simulink model "single_phase_multilevel"  (R2025a)
settings: Solver=ode1be  StartTime=0.0  StopTime=simlength  FixedStep=tc  RelTol=1e-3
values from neighbouring files (symbols this model uses):
  Vfc1_base = Udc/5    [plotting_results.m]    (also in plotting_results_hf.m)
  Vfc2_base = 2*Vfc1_base    [plotting_results.m]    (also in plotting_results_hf.m)
  Vfc3_base = 3*Vfc1_base    [plotting_results.m]    (also in plotting_results_hf.m)
  Vfc4_base = 4*Vfc1_base    [plotting_results.m]    (also in plotting_results_hf.m)
undefined symbols (not defined in the file or in its folder): DThs_init, g0_4Hz, g1_4Hz, I_FS, kalman_omega, kalman_theta, ki_i_inv, ki_v_inv, kp_i_inv, kp_v_inv, Lconn, LFu1, m_dead_time, m_duty_open_loop, magnitude, n1, n10, omega_ref, phase_shift_mod11, phase_shift_mod21, phase_shift_mod31, phase_shift_mod41, phase_shift_mod51, precharge_off, q1kalman, q2kalman, Rbalance, Rconn, RFu, Rg_off, Rg_on, Rkalman, RLFu1, Rprecharge, Tambient, tc, time_pwm_enable, tPWM, ts, V_FS, VCFc_5_init, Vgate_base, weigth
libraries: fl_lib x281, nesl_utility x97, ee_lib x15, simulink x1
(part 2 of 6)

== system single_phase_multilevel/flying_capacitor_leg/fc1 ==
  CFc_1 : fl_lib/Electrical/Electrical Elements/Capacitor  c=CFc_1 F  r=1e-6 Ohm  g=0 1/Ohm  i_specify=off  i_priority=None  i=0 A  i_nominal_specify=off  i_nominal_value=1  i_nominal_unit=A  v_specify=off  v_priority=None  v=0 V  v_nominal_specify=off  v_nominal_value=1  v_nominal_unit=V  vc_specify=on  vc_priority=High  vc=VCFc_1_init V  vc_nominal_specify=off  vc_nominal_value=1  vc_nominal_unit=V
  CFi_HF_1 : fl_lib/Electrical/Electrical Elements/Capacitor  c=CFi_HF_1 F  r=1e-6 Ohm  g=0 1/Ohm  i_specify=off  i_priority=None  i=0 A  i_nominal_specify=off  i_nominal_value=1  i_nominal_unit=A  v_specify=off  v_priority=None  v=0 V  v_nominal_specify=off  v_nominal_value=1  v_nominal_unit=V  vc_specify=on  vc_priority=High  vc=VCFc_1_init V  vc_nominal_specify=off  vc_nominal_value=1  vc_nominal_unit=V
  Current Sensor : fl_lib/Electrical/Electrical Sensors/Current Sensor
  Current Sensor1 : fl_lib/Electrical/Electrical Sensors/Current Sensor
  LCFc_1 : fl_lib/Electrical/Electrical Elements/Inductor  l=LCFc_1 H  r=RCFc_1 Ohm  g=1e-9 1/Ohm  i_specify=off  i_priority=None  i=0 A  i_nominal_specify=off  i_nominal_value=1  i_nominal_unit=A  v_specify=off  v_priority=None  v=0 V  v_nominal_specify=off  v_nominal_value=1  v_nominal_unit=V  i_L_specify=off  i_L_priority=High  i_L=0 A  i_L_nominal_specify=off  i_L_nominal_value=1  i_L_nominal_unit=A
  LCFi_HF_1 : fl_lib/Electrical/Electrical Elements/Inductor  l=LCFi_HF_1 H  r=RCFi_HF_1 Ohm  g=1e-9 1/Ohm  i_specify=off  i_priority=None  i=0 A  i_nominal_specify=off  i_nominal_value=1  i_nominal_unit=A  v_specify=off  v_priority=None  v=0 V  v_nominal_specify=off  v_nominal_value=1  v_nominal_unit=V  i_L_specify=off  i_L_priority=High  i_L=0 A  i_L_nominal_specify=off  i_L_nominal_value=1  i_L_nominal_unit=A
  PS-Simulink Converter : nesl_utility/PS-Simulink Converter  PhysicalDomain=network_engine_domain  SubClassName=ps_output  LeftPortType=input  RightPortType=output  PseudoPeriodic=off  Frequencies=[]  VectorFormat=1-D array  Unit=A  AffineConversion=off
  PS-Simulink Converter1 : nesl_utility/PS-Simulink Converter  PhysicalDomain=network_engine_domain  SubClassName=ps_output  LeftPortType=input  RightPortType=output  PseudoPeriodic=off  Frequencies=[]  VectorFormat=1-D array  Unit=V  AffineConversion=off
  PS-Simulink Converter2 : nesl_utility/PS-Simulink Converter  PhysicalDomain=network_engine_domain  SubClassName=ps_output  LeftPortType=input  RightPortType=output  PseudoPeriodic=off  Frequencies=[]  VectorFormat=1-D array  Unit=A  AffineConversion=off
  Voltage Sensor : fl_lib/Electrical/Electrical Sensors/Voltage Sensor
  1 : PMIOPort  Side=Left
  2 : PMIOPort  Port=2  Side=Right
  tag scope: current_flying_capacitor_1=global, current_hf_capacitor_1=global, voltage_flying_capacitor_1=global
  wires:
  PS-Simulink Converter1/1 -> [voltage_flying_capacitor_1]
  PS-Simulink Converter/1 -> [current_flying_capacitor_1]
  PS-Simulink Converter2/1 -> [current_hf_capacitor_1]
  connections:
  Current Sensor/RConn2 -- CFc_1/LConn1
  Voltage Sensor/RConn2 -- 2/RConn1 -- LCFi_HF_1/RConn1 -- LCFc_1/RConn1
  Voltage Sensor/RConn1 -- PS-Simulink Converter1/LConn1
  Current Sensor/RConn1 -- PS-Simulink Converter/LConn1
  Current Sensor/LConn1 -- Current Sensor1/LConn1 -- 1/RConn1 -- Voltage Sensor/LConn1
  LCFc_1/LConn1 -- CFc_1/RConn1
  CFi_HF_1/RConn1 -- LCFi_HF_1/LConn1
  Current Sensor1/RConn2 -- CFi_HF_1/LConn1
  Current Sensor1/RConn1 -- PS-Simulink Converter2/LConn1

== system single_phase_multilevel/flying_capacitor_leg/fc2 ==
  CFc_2 : fl_lib/Electrical/Electrical Elements/Capacitor  c=CFc_2 F  r=1e-6 Ohm  g=0 1/Ohm  i_specify=off  i_priority=None  i=0 A  i_nominal_specify=off  i_nominal_value=1  i_nominal_unit=A  v_specify=off  v_priority=None  v=0 V  v_nominal_specify=off  v_nominal_value=1  v_nominal_unit=V  vc_specify=on  vc_priority=High  vc=VCFc_2_init V  vc_nominal_specify=off  vc_nominal_value=1  vc_nominal_unit=V
  CFi_HF_2 : fl_lib/Electrical/Electrical Elements/Capacitor  c=CFi_HF_2 F  r=1e-6 Ohm  g=0 1/Ohm  i_specify=off  i_priority=None  i=0 A  i_nominal_specify=off  i_nominal_value=1  i_nominal_unit=A  v_specify=off  v_priority=None  v=0 V  v_nominal_specify=off  v_nominal_value=1  v_nominal_unit=V  vc_specify=on  vc_priority=High  vc=VCFc_2_init V  vc_nominal_specify=off  vc_nominal_value=1  vc_nominal_unit=V
  Current Sensor : fl_lib/Electrical/Electrical Sensors/Current Sensor
  LCFc_2 : fl_lib/Electrical/Electrical Elements/Inductor  l=LCFc_2 H  r=RCFc_2 Ohm  g=1e-9 1/Ohm  i_specify=off  i_priority=None  i=0 A  i_nominal_specify=off  i_nominal_value=1  i_nominal_unit=A  v_specify=off  v_priority=None  v=0 V  v_nominal_specify=off  v_nominal_value=1  v_nominal_unit=V  i_L_specify=off  i_L_priority=High  i_L=0 A  i_L_nominal_specify=off  i_L_nominal_value=1  i_L_nominal_unit=A
  LCFi_HF_2 : fl_lib/Electrical/Electrical Elements/Inductor  l=LCFi_HF_2 H  r=RCFi_HF_2 Ohm  g=1e-9 1/Ohm  i_specify=off  i_priority=None  i=0 A  i_nominal_specify=off  i_nominal_value=1  i_nominal_unit=A  v_specify=off  v_priority=None  v=0 V  v_nominal_specify=off  v_nominal_value=1  v_nominal_unit=V  i_L_specify=off  i_L_priority=High  i_L=0 A  i_L_nominal_specify=off  i_L_nominal_value=1  i_L_nominal_unit=A
  PS-Simulink Converter : nesl_utility/PS-Simulink Converter  PhysicalDomain=network_engine_domain  SubClassName=ps_output  LeftPortType=input  RightPortType=output  PseudoPeriodic=off  Frequencies=[]  VectorFormat=1-D array  Unit=A  AffineConversion=off
  PS-Simulink Converter2 : nesl_utility/PS-Simulink Converter  PhysicalDomain=network_engine_domain  SubClassName=ps_output  LeftPortType=input  RightPortType=output  PseudoPeriodic=off  Frequencies=[]  VectorFormat=1-D array  Unit=V  AffineConversion=off
  Voltage Sensor1 : fl_lib/Electrical/Electrical Sensors/Voltage Sensor
  1 : PMIOPort  Side=Left
  2 : PMIOPort  Port=2  Side=Right
  tag scope: current_flying_capacitor_2=global, voltage_flying_capacitor_2=global
  wires:
  PS-Simulink Converter2/1 -> [voltage_flying_capacitor_2]
  PS-Simulink Converter/1 -> [current_flying_capacitor_2]
  connections:
  Voltage Sensor1/RConn2 -- LCFi_HF_2/RConn1 -- Current Sensor/RConn2 -- 2/RConn1
  Voltage Sensor1/LConn1 -- CFi_HF_2/LConn1 -- CFc_2/LConn1 -- 1/RConn1
  Voltage Sensor1/RConn1 -- PS-Simulink Converter2/LConn1
  Current Sensor/RConn1 -- PS-Simulink Converter/LConn1
  LCFc_2/LConn1 -- CFc_2/RConn1
  Current Sensor/LConn1 -- LCFc_2/RConn1
  LCFi_HF_2/LConn1 -- CFi_HF_2/RConn1

== system single_phase_multilevel/flying_capacitor_leg/fc3 ==
  CFc_3 : fl_lib/Electrical/Electrical Elements/Capacitor  c=CFc_3 F  r=1e-6 Ohm  g=0 1/Ohm  i_specify=off  i_priority=None  i=0 A  i_nominal_specify=off  i_nominal_value=1  i_nominal_unit=A  v_specify=off  v_priority=None  v=0 V  v_nominal_specify=off  v_nominal_value=1  v_nominal_unit=V  vc_specify=on  vc_priority=High  vc=VCFc_3_init V  vc_nominal_specify=off  vc_nominal_value=1  vc_nominal_unit=V
  CFi_HF_3 : fl_lib/Electrical/Electrical Elements/Capacitor  c=CFi_HF_3 F  r=1e-6 Ohm  g=0 1/Ohm  i_specify=off  i_priority=None  i=0 A  i_nominal_specify=off  i_nominal_value=1  i_nominal_unit=A  v_specify=off  v_priority=None  v=0 V  v_nominal_specify=off  v_nominal_value=1  v_nominal_unit=V  vc_specify=on  vc_priority=High  vc=VCFc_3_init V  vc_nominal_specify=off  vc_nominal_value=1  vc_nominal_unit=V
  Current Sensor : fl_lib/Electrical/Electrical Sensors/Current Sensor
  LCFc_3 : fl_lib/Electrical/Electrical Elements/Inductor  l=LCFc_3 H  r=RCFc_3 Ohm  g=1e-9 1/Ohm  i_specify=off  i_priority=None  i=0 A  i_nominal_specify=off  i_nominal_value=1  i_nominal_unit=A  v_specify=off  v_priority=None  v=0 V  v_nominal_specify=off  v_nominal_value=1  v_nominal_unit=V  i_L_specify=off  i_L_priority=High  i_L=0 A  i_L_nominal_specify=off  i_L_nominal_value=1  i_L_nominal_unit=A
  LCFi_HF_3 : fl_lib/Electrical/Electrical Elements/Inductor  l=LCFi_HF_3 H  r=RCFi_HF_3 Ohm  g=1e-9 1/Ohm  i_specify=off  i_priority=None  i=0 A  i_nominal_specify=off  i_nominal_value=1  i_nominal_unit=A  v_specify=off  v_priority=None  v=0 V  v_nominal_specify=off  v_nominal_value=1  v_nominal_unit=V  i_L_specify=off  i_L_priority=High  i_L=0 A  i_L_nominal_specify=off  i_L_nominal_value=1  i_L_nominal_unit=A
  PS-Simulink Converter : nesl_utility/PS-Simulink Converter  PhysicalDomain=network_engine_domain  SubClassName=ps_output  LeftPortType=input  RightPortType=output  PseudoPeriodic=off  Frequencies=[]  VectorFormat=1-D array  Unit=A  AffineConversion=off
  PS-Simulink Converter2 : nesl_utility/PS-Simulink Converter  PhysicalDomain=network_engine_domain  SubClassName=ps_output  LeftPortType=input  RightPortType=output  PseudoPeriodic=off  Frequencies=[]  VectorFormat=1-D array  Unit=V  AffineConversion=off
  Voltage Sensor1 : fl_lib/Electrical/Electrical Sensors/Voltage Sensor
  1 : PMIOPort  Side=Left
  2 : PMIOPort  Port=2  Side=Right
  tag scope: current_flying_capacitor_3=global, voltage_flying_capacitor_3=global
  wires:
  PS-Simulink Converter2/1 -> [voltage_flying_capacitor_3]
  PS-Simulink Converter/1 -> [current_flying_capacitor_3]
  connections:
  CFc_3/LConn1 -- CFi_HF_3/LConn1 -- Voltage Sensor1/LConn1 -- 1/RConn1
  Voltage Sensor1/RConn1 -- PS-Simulink Converter2/LConn1
  Voltage Sensor1/RConn2 -- LCFi_HF_3/RConn1 -- Current Sensor/RConn2 -- 2/RConn1
  Current Sensor/RConn1 -- PS-Simulink Converter/LConn1
  LCFc_3/LConn1 -- CFc_3/RConn1
  Current Sensor/LConn1 -- LCFc_3/RConn1
  LCFi_HF_3/LConn1 -- CFi_HF_3/RConn1

== system single_phase_multilevel/flying_capacitor_leg/fc4 ==
  CFc_4 : fl_lib/Electrical/Electrical Elements/Capacitor  c=CFc_4 F  r=1e-6 Ohm  g=0 1/Ohm  i_specify=off  i_priority=None  i=0 A  i_nominal_specify=off  i_nominal_value=1  i_nominal_unit=A  v_specify=off  v_priority=None  v=0 V  v_nominal_specify=off  v_nominal_value=1  v_nominal_unit=V  vc_specify=on  vc_priority=High  vc=VCFc_4_init V  vc_nominal_specify=off  vc_nominal_value=1  vc_nominal_unit=V
  CFi_HF_4 : fl_lib/Electrical/Electrical Elements/Capacitor  c=CFi_HF_4 F  r=1e-6 Ohm  g=0 1/Ohm  i_specify=off  i_priority=None  i=0 A  i_nominal_specify=off  i_nominal_value=1  i_nominal_unit=A  v_specify=off  v_priority=None  v=0 V  v_nominal_specify=off  v_nominal_value=1  v_nominal_unit=V  vc_specify=on  vc_priority=High  vc=VCFc_4_init V  vc_nominal_specify=off  vc_nominal_value=1  vc_nominal_unit=V
  Current Sensor : fl_lib/Electrical/Electrical Sensors/Current Sensor
  LCFc_4 : fl_lib/Electrical/Electrical Elements/Inductor  l=LCFc_4 H  r=RCFc_4 Ohm  g=1e-9 1/Ohm  i_specify=off  i_priority=None  i=0 A  i_nominal_specify=off  i_nominal_value=1  i_nominal_unit=A  v_specify=off  v_priority=None  v=0 V  v_nominal_specify=off  v_nominal_value=1  v_nominal_unit=V  i_L_specify=off  i_L_priority=High  i_L=0 A  i_L_nominal_specify=off  i_L_nominal_value=1  i_L_nominal_unit=A
  LCFi_HF_4 : fl_lib/Electrical/Electrical Elements/Inductor  l=LCFi_HF_4 H  r=RCFi_HF_4 Ohm  g=1e-9 1/Ohm  i_specify=off  i_priority=None  i=0 A  i_nominal_specify=off  i_nominal_value=1  i_nominal_unit=A  v_specify=off  v_priority=None  v=0 V  v_nominal_specify=off  v_nominal_value=1  v_nominal_unit=V  i_L_specify=off  i_L_priority=High  i_L=0 A  i_L_nominal_specify=off  i_L_nominal_value=1  i_L_nominal_unit=A
  PS-Simulink Converter : nesl_utility/PS-Simulink Converter  PhysicalDomain=network_engine_domain  SubClassName=ps_output  LeftPortType=input  RightPortType=output  PseudoPeriodic=off  Frequencies=[]  VectorFormat=1-D array  Unit=A  AffineConversion=off
  PS-Simulink Converter2 : nesl_utility/PS-Simulink Converter  PhysicalDomain=network_engine_domain  SubClassName=ps_output  LeftPortType=input  RightPortType=output  PseudoPeriodic=off  Frequencies=[]  VectorFormat=1-D array  Unit=V  AffineConversion=off
  Voltage Sensor1 : fl_lib/Electrical/Electrical Sensors/Voltage Sensor
  1 : PMIOPort  Side=Left
  2 : PMIOPort  Port=2  Side=Right
  tag scope: current_flying_capacitor_4=global, voltage_flying_capacitor_4=global
  wires:
  PS-Simulink Converter2/1 -> [voltage_flying_capacitor_4]
  PS-Simulink Converter/1 -> [current_flying_capacitor_4]
  connections:
  Voltage Sensor1/LConn1 -- CFi_HF_4/LConn1 -- CFc_4/LConn1 -- 1/RConn1
  Voltage Sensor1/RConn1 -- PS-Simulink Converter2/LConn1
  Voltage Sensor1/RConn2 -- LCFi_HF_4/RConn1 -- Current Sensor/RConn2 -- 2/RConn1
  Current Sensor/RConn1 -- PS-Simulink Converter/LConn1
  Current Sensor/LConn1 -- LCFc_4/RConn1
  LCFc_4/LConn1 -- CFc_4/RConn1
  LCFi_HF_4/LConn1 -- CFi_HF_4/RConn1

== system single_phase_multilevel/flying_capacitor_leg/fc51 ==
  CFc_51 : fl_lib/Electrical/Electrical Elements/Capacitor  c=CFc_51 F  r=1e-6 Ohm  g=0 1/Ohm  i_specify=off  i_priority=None  i=0 A  i_nominal_specify=off  i_nominal_value=1  i_nominal_unit=A  v_specify=off  v_priority=None  v=0 V  v_nominal_specify=off  v_nominal_value=1  v_nominal_unit=V  vc_specify=on  vc_priority=High  vc=VCFc_5_init/2 V  vc_nominal_specify=off  vc_nominal_value=1  vc_nominal_unit=V
  Current Sensor : fl_lib/Electrical/Electrical Sensors/Current Sensor
  LCFc_51 : fl_lib/Electrical/Electrical Elements/Inductor  l=LCFc_51 H  r=RCFc_51 Ohm  g=1e-9 1/Ohm  i_specify=off  i_priority=None  i=0 A  i_nominal_specify=off  i_nominal_value=1  i_nominal_unit=A  v_specify=off  v_priority=None  v=0 V  v_nominal_specify=off  v_nominal_value=1  v_nominal_unit=V  i_L_specify=off  i_L_priority=High  i_L=0 A  i_L_nominal_specify=off  i_L_nominal_value=1  i_L_nominal_unit=A
  PS-Simulink Converter : nesl_utility/PS-Simulink Converter  PhysicalDomain=network_engine_domain  SubClassName=ps_output  LeftPortType=input  RightPortType=output  PseudoPeriodic=off  Frequencies=[]  VectorFormat=1-D array  Unit=A  AffineConversion=off
  PS-Simulink Converter2 : nesl_utility/PS-Simulink Converter  PhysicalDomain=network_engine_domain  SubClassName=ps_output  LeftPortType=input  RightPortType=output  PseudoPeriodic=off  Frequencies=[]  VectorFormat=1-D array  Unit=V  AffineConversion=off
  Voltage Sensor1 : fl_lib/Electrical/Electrical Sensors/Voltage Sensor
  1 : PMIOPort  Side=Left
  2 : PMIOPort  Port=2  Side=Right
  tag scope: current_flying_capacitor_51=global, voltage_flying_capacitor_51=global
  wires:
  PS-Simulink Converter/1 -> [current_flying_capacitor_51]
  PS-Simulink Converter2/1 -> [voltage_flying_capacitor_51]
  connections:
  CFc_51/LConn1 -- Voltage Sensor1/LConn1 -- 1/RConn1
  Current Sensor/RConn1 -- PS-Simulink Converter/LConn1
  LCFc_51/LConn1 -- CFc_51/RConn1
  Current Sensor/RConn2 -- Voltage Sensor1/RConn2 -- 2/RConn1
  Current Sensor/LConn1 -- LCFc_51/RConn1
  Voltage Sensor1/RConn1 -- PS-Simulink Converter2/LConn1

== system single_phase_multilevel/flying_capacitor_leg/fc52 ==
  CFc_52 : fl_lib/Electrical/Electrical Elements/Capacitor  c=CFc_52 F  r=1e-6 Ohm  g=0 1/Ohm  i_specify=off  i_priority=None  i=0 A  i_nominal_specify=off  i_nominal_value=1  i_nominal_unit=A  v_specify=off  v_priority=None  v=0 V  v_nominal_specify=off  v_nominal_value=1  v_nominal_unit=V  vc_specify=on  vc_priority=High  vc=VCFc_5_init/2 V  vc_nominal_specify=off  vc_nominal_value=1  vc_nominal_unit=V
  Current Sensor : fl_lib/Electrical/Electrical Sensors/Current Sensor
  LCFc_52 : fl_lib/Electrical/Electrical Elements/Inductor  l=LCFc_52 H  r=RCFc_52 Ohm  g=1e-9 1/Ohm  i_specify=off  i_priority=None  i=0 A  i_nominal_specify=off  i_nominal_value=1  i_nominal_unit=A  v_specify=off  v_priority=None  v=0 V  v_nominal_specify=off  v_nominal_value=1  v_nominal_unit=V  i_L_specify=off  i_L_priority=High  i_L=0 A  i_L_nominal_specify=off  i_L_nominal_value=1  i_L_nominal_unit=A
  PS-Simulink Converter : nesl_utility/PS-Simulink Converter  PhysicalDomain=network_engine_domain  SubClassName=ps_output  LeftPortType=input  RightPortType=output  PseudoPeriodic=off  Frequencies=[]  VectorFormat=1-D array  Unit=A  AffineConversion=off
  PS-Simulink Converter2 : nesl_utility/PS-Simulink Converter  PhysicalDomain=network_engine_domain  SubClassName=ps_output  LeftPortType=input  RightPortType=output  PseudoPeriodic=off  Frequencies=[]  VectorFormat=1-D array  Unit=V  AffineConversion=off
  Voltage Sensor1 : fl_lib/Electrical/Electrical Sensors/Voltage Sensor
  1 : PMIOPort  Side=Left
  2 : PMIOPort  Port=2  Side=Right
  tag scope: current_flying_capacitor_52=global, voltage_flying_capacitor_52=global
  wires:
  PS-Simulink Converter/1 -> [current_flying_capacitor_52]
  PS-Simulink Converter2/1 -> [voltage_flying_capacitor_52]
  connections:
  CFc_52/LConn1 -- Voltage Sensor1/LConn1 -- 1/RConn1
  Current Sensor/RConn1 -- PS-Simulink Converter/LConn1
  LCFc_52/LConn1 -- CFc_52/RConn1
  Current Sensor/RConn2 -- Voltage Sensor1/RConn2 -- 2/RConn1
  Current Sensor/LConn1 -- LCFc_52/RConn1
  Voltage Sensor1/RConn1 -- PS-Simulink Converter2/LConn1

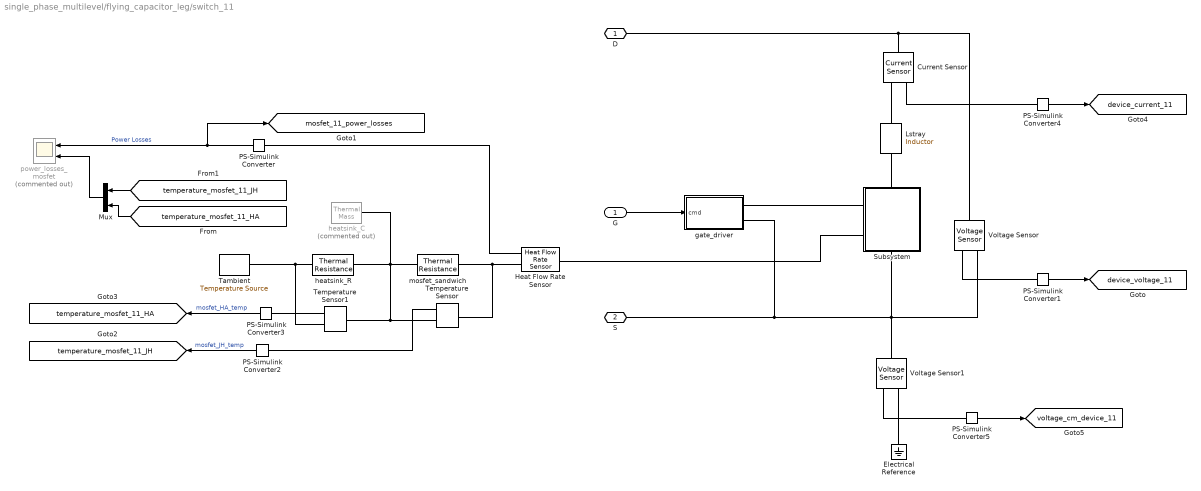
== system single_phase_multilevel/flying_capacitor_leg/switch_11 ==
  G : Inport
  Current Sensor : fl_lib/Electrical/Electrical Sensors/Current Sensor
  Electrical Reference : fl_lib/Electrical/Electrical Elements/Electrical Reference
  Heat Flow Rate Sensor : fl_lib/Thermal/Thermal Sensors/Heat Flow Rate Sensor
  Lstray : fl_lib/Electrical/Electrical Elements/Inductor  l=Lstray H  r=0 Ohm  g=1e-9 1/Ohm  i_specify=off  i_priority=None  i=0 A  i_nominal_specify=off  i_nominal_value=1  i_nominal_unit=A  v_specify=off  v_priority=None  v=0 V  v_nominal_specify=off  v_nominal_value=1  v_nominal_unit=V  i_L_specify=off  i_L_priority=High  i_L=0 A  i_L_nominal_specify=off  i_L_nominal_value=1  i_L_nominal_unit=A
  Mux : Mux  Inputs=2
  PS-Simulink Converter : nesl_utility/PS-Simulink Converter  PhysicalDomain=network_engine_domain  SubClassName=ps_output  LeftPortType=input  RightPortType=output  PseudoPeriodic=off  Frequencies=[]  VectorFormat=1-D array  Unit=W  AffineConversion=off
  PS-Simulink Converter1 : nesl_utility/PS-Simulink Converter  PhysicalDomain=network_engine_domain  SubClassName=ps_output  LeftPortType=input  RightPortType=output  PseudoPeriodic=off  Frequencies=[]  VectorFormat=1-D array  Unit=V  AffineConversion=off
  PS-Simulink Converter2 : nesl_utility/PS-Simulink Converter  PhysicalDomain=network_engine_domain  SubClassName=ps_output  LeftPortType=input  RightPortType=output  PseudoPeriodic=off  Frequencies=[]  VectorFormat=1-D array  Unit=degC  AffineConversion=off
  PS-Simulink Converter3 : nesl_utility/PS-Simulink Converter  PhysicalDomain=network_engine_domain  SubClassName=ps_output  LeftPortType=input  RightPortType=output  PseudoPeriodic=off  Frequencies=[]  VectorFormat=1-D array  Unit=degC  AffineConversion=off
  PS-Simulink Converter4 : nesl_utility/PS-Simulink Converter  PhysicalDomain=network_engine_domain  SubClassName=ps_output  LeftPortType=input  RightPortType=output  PseudoPeriodic=off  Frequencies=[]  VectorFormat=1-D array  Unit=A  AffineConversion=off
  PS-Simulink Converter5 : nesl_utility/PS-Simulink Converter  PhysicalDomain=network_engine_domain  SubClassName=ps_output  LeftPortType=input  RightPortType=output  PseudoPeriodic=off  Frequencies=[]  VectorFormat=1-D array  Unit=V  AffineConversion=off
  Subsystem : Subsystem
      settings: PortSchema="{\"entries\":[{\"content\":{\"sides\":[{\"content\":{\"connectorIds\":[\"LConn1\",\"LConn2\"]},\"type\":\"ConnectorPlacement.EquallySpacedRectSide\",\"uuid\":\"6f524266-aba9-462a-9d72-1145635a1e26\"},{\"content\":{\"side\":\"RIGHT\"},\"type\":\"ConnectorPlacement.EquallySpacedRectSide\",\"uuid\":\"542b2524-63ec-4375-9435-097c03e43763\"},{\"content\":{\"connectorIds\":[\"LConn3\"],\"side\":\"TOP\"},\"type\":\"ConnectorPlacement.EquallySpacedRectSide\",\"uuid\":\"19216a12-d28e-49a5-8583-2c9307a52e67\"},{\"content\":{\"connectorIds\":[\"RConn1\"],\"side\":\"BOTTOM\"},\"type\":\"ConnectorPlacement.EquallySpacedRectSide\",\"uuid\":\"0f3a6771-cb7b-4dcc-bba9-376db372f9ba\"}]},\"type\":\"ConnectorPlacement.EquallySpacedConnector\",\"uuid\":\"2de64d24-c5c0-4ec1-b56f-991356417e7b\"}],\"packageUris\":[\"http://schema.mathworks.com/mf0/Connector/R2020b\"],\"version\":\"1.0\"}"
  Tambient : fl_lib/Thermal/Thermal Sources/Temperature Source  temperature=Tambient degC
  Temperature Sensor : fl_lib/Thermal/Thermal Sensors/Temperature Sensor  temperature_measure=foundation.enum.MeasurementReference.difference
  Temperature Sensor1 : fl_lib/Thermal/Thermal Sensors/Temperature Sensor  temperature_measure=foundation.enum.MeasurementReference.difference
  Voltage Sensor : fl_lib/Electrical/Electrical Sensors/Voltage Sensor
  Voltage Sensor1 : fl_lib/Electrical/Electrical Sensors/Voltage Sensor
  gate_driver : Subsystem
  heatsink_C : fl_lib/Thermal/Thermal Elements/Thermal Mass  Commented=on  mass_type=foundation.enum.constant_variable.constant  mass=weigth/6 kg  sp_heat=cp_al J/(K*kg)  mass_min=1e-6 kg  num_ports=foundation.enum.numPorts2.one  m_specify=off  m_priority=High  m=1 kg  m_nominal_specify=off  m_nominal_value=1  m_nominal_unit=kg  T_specify=on  T_priority=High  T=DThs_init+Tambient degC  T_nominal_specify=off  T_nominal_value=1  T_nominal_unit=K  Q_specify=off  Q_priority=High  Q=0 W  Q_nominal_specify=off  Q_nominal_value=1  Q_nominal_unit=W
  heatsink_R : fl_lib/Thermal/Thermal Elements/Thermal Resistance  resistance=Rth_mosfet_HA K/W  T_specify=off  T_priority=High  T=0 deltadegC  T_nominal_specify=off  T_nominal_value=1  T_nominal_unit=K  Q_specify=off  Q_priority=None  Q=0 W  Q_nominal_specify=off  Q_nominal_value=1  Q_nominal_unit=W
  mosfet_sandwich : fl_lib/Thermal/Thermal Elements/Thermal Resistance  resistance=Rth_mosfet_JH K/W  T_specify=off  T_priority=High  T=0 degC  T_nominal_specify=off  T_nominal_value=1  T_nominal_unit=K  Q_specify=off  Q_priority=None  Q=0 W  Q_nominal_specify=off  Q_nominal_value=1  Q_nominal_unit=W
  power_losses_mosfet : Scope  Commented=on  NumInputPorts=2
      settings: SampleTime=tc  ActiveDisplayYMinimum=-6.15902  ActiveDisplayYMaximum=55.43118
  D : PMIOPort  Side=Left
  S : PMIOPort  Port=2  Side=Right
  tag scope: device_current_11=global, device_voltage_11=global, mosfet_11_power_losses=global, temperature_mosfet_11_HA=global, temperature_mosfet_11_JH=global, voltage_cm_device_11=global
  wires:
  PS-Simulink Converter1/1 -> [device_voltage_11]
  Mux/1 -> power_losses_mosfet/2
  PS-Simulink Converter3/1 -> [temperature_mosfet_11_HA]  "mosfet_HA_temp"
  [temperature_mosfet_11_JH] -> Mux/1
  [temperature_mosfet_11_HA] -> Mux/2
  PS-Simulink Converter2/1 -> [temperature_mosfet_11_JH]  "mosfet_JH_temp"
  PS-Simulink Converter/1 -> power_losses_mosfet/1, [mosfet_11_power_losses]  "Power Losses"
  PS-Simulink Converter4/1 -> [device_current_11]
  PS-Simulink Converter5/1 -> [voltage_cm_device_11]
  G/1 -> gate_driver/1(cmd)
  connections:
  Voltage Sensor/RConn1 -- PS-Simulink Converter1/LConn1
  Heat Flow Rate Sensor/RConn2 -- mosfet_sandwich/LConn1 -- Temperature Sensor/LConn1
  Temperature Sensor1/RConn1 -- heatsink_R/RConn1 -- Tambient/LConn1
  Temperature Sensor1/LConn1 -- Temperature Sensor/RConn1 -- heatsink_R/LConn1 -- heatsink_C/LConn1 -- mosfet_sandwich/RConn1
  Temperature Sensor1/RConn2 -- PS-Simulink Converter3/LConn1
  Temperature Sensor/RConn2 -- PS-Simulink Converter2/LConn1
  Voltage Sensor/RConn2 -- Voltage Sensor1/LConn1 -- Subsystem/RConn1 -- S/RConn1 -- gate_driver/RConn2
  PS-Simulink Converter/LConn1 -- Heat Flow Rate Sensor/RConn1
  Current Sensor/LConn1 -- D/RConn1 -- Voltage Sensor/LConn1
  Current Sensor/RConn1 -- PS-Simulink Converter4/LConn1
  PS-Simulink Converter5/LConn1 -- Voltage Sensor1/RConn1
  Voltage Sensor1/RConn2 -- Electrical Reference/LConn1
  Lstray/LConn1 -- Current Sensor/RConn2
  Subsystem/LConn3 -- Lstray/RConn1
  Heat Flow Rate Sensor/LConn1 -- Subsystem/LConn2
  Subsystem/LConn1 -- gate_driver/RConn1

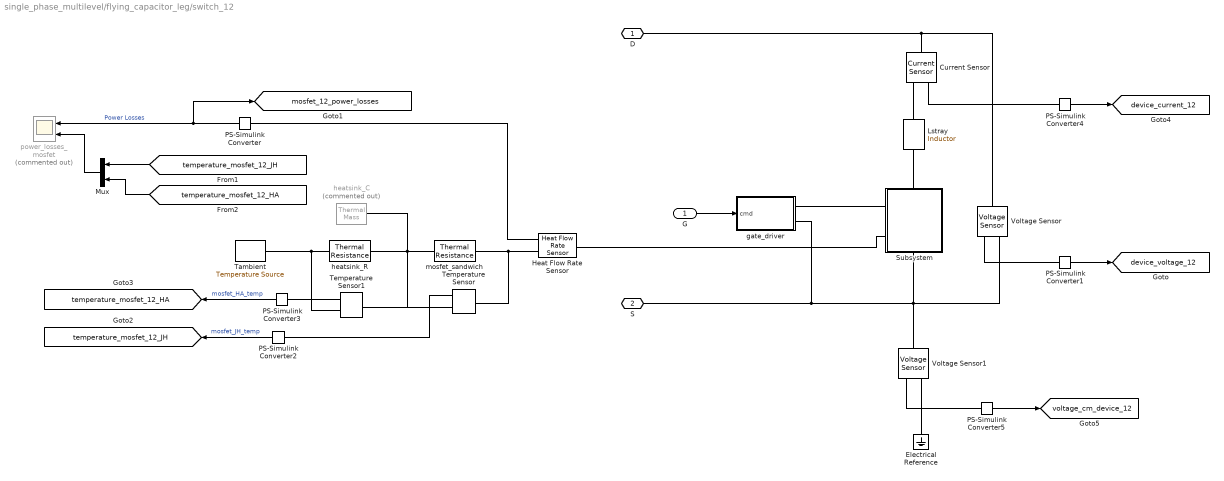
== system single_phase_multilevel/flying_capacitor_leg/switch_12 ==
  G : Inport
  Current Sensor : fl_lib/Electrical/Electrical Sensors/Current Sensor
  Electrical Reference : fl_lib/Electrical/Electrical Elements/Electrical Reference
  Heat Flow Rate Sensor : fl_lib/Thermal/Thermal Sensors/Heat Flow Rate Sensor
  Lstray : fl_lib/Electrical/Electrical Elements/Inductor  l=Lstray H  r=0 Ohm  g=1e-9 1/Ohm  i_specify=off  i_priority=None  i=0 A  i_nominal_specify=off  i_nominal_value=1  i_nominal_unit=A  v_specify=off  v_priority=None  v=0 V  v_nominal_specify=off  v_nominal_value=1  v_nominal_unit=V  i_L_specify=off  i_L_priority=High  i_L=0 A  i_L_nominal_specify=off  i_L_nominal_value=1  i_L_nominal_unit=A
  Mux : Mux  Inputs=2
  PS-Simulink Converter : nesl_utility/PS-Simulink Converter  PhysicalDomain=network_engine_domain  SubClassName=ps_output  LeftPortType=input  RightPortType=output  PseudoPeriodic=off  Frequencies=[]  VectorFormat=1-D array  Unit=W  AffineConversion=off
  PS-Simulink Converter1 : nesl_utility/PS-Simulink Converter  PhysicalDomain=network_engine_domain  SubClassName=ps_output  LeftPortType=input  RightPortType=output  PseudoPeriodic=off  Frequencies=[]  VectorFormat=1-D array  Unit=V  AffineConversion=off
  PS-Simulink Converter2 : nesl_utility/PS-Simulink Converter  PhysicalDomain=network_engine_domain  SubClassName=ps_output  LeftPortType=input  RightPortType=output  PseudoPeriodic=off  Frequencies=[]  VectorFormat=1-D array  Unit=degC  AffineConversion=off
  PS-Simulink Converter3 : nesl_utility/PS-Simulink Converter  PhysicalDomain=network_engine_domain  SubClassName=ps_output  LeftPortType=input  RightPortType=output  PseudoPeriodic=off  Frequencies=[]  VectorFormat=1-D array  Unit=degC  AffineConversion=off
  PS-Simulink Converter4 : nesl_utility/PS-Simulink Converter  PhysicalDomain=network_engine_domain  SubClassName=ps_output  LeftPortType=input  RightPortType=output  PseudoPeriodic=off  Frequencies=[]  VectorFormat=1-D array  Unit=A  AffineConversion=off
  PS-Simulink Converter5 : nesl_utility/PS-Simulink Converter  PhysicalDomain=network_engine_domain  SubClassName=ps_output  LeftPortType=input  RightPortType=output  PseudoPeriodic=off  Frequencies=[]  VectorFormat=1-D array  Unit=V  AffineConversion=off
  Subsystem : Subsystem
      settings: PortSchema="{\"entries\":[{\"content\":{\"sides\":[{\"content\":{\"connectorIds\":[\"LConn1\",\"LConn2\"]},\"type\":\"ConnectorPlacement.EquallySpacedRectSide\",\"uuid\":\"6f524266-aba9-462a-9d72-1145635a1e26\"},{\"content\":{\"side\":\"RIGHT\"},\"type\":\"ConnectorPlacement.EquallySpacedRectSide\",\"uuid\":\"542b2524-63ec-4375-9435-097c03e43763\"},{\"content\":{\"connectorIds\":[\"LConn3\"],\"side\":\"TOP\"},\"type\":\"ConnectorPlacement.EquallySpacedRectSide\",\"uuid\":\"19216a12-d28e-49a5-8583-2c9307a52e67\"},{\"content\":{\"connectorIds\":[\"RConn1\"],\"side\":\"BOTTOM\"},\"type\":\"ConnectorPlacement.EquallySpacedRectSide\",\"uuid\":\"0f3a6771-cb7b-4dcc-bba9-376db372f9ba\"}]},\"type\":\"ConnectorPlacement.EquallySpacedConnector\",\"uuid\":\"2de64d24-c5c0-4ec1-b56f-991356417e7b\"}],\"packageUris\":[\"http://schema.mathworks.com/mf0/Connector/R2020b\"],\"version\":\"1.0\"}"
  Tambient : fl_lib/Thermal/Thermal Sources/Temperature Source  temperature=Tambient degC
  Temperature Sensor : fl_lib/Thermal/Thermal Sensors/Temperature Sensor  temperature_measure=foundation.enum.MeasurementReference.difference
  Temperature Sensor1 : fl_lib/Thermal/Thermal Sensors/Temperature Sensor  temperature_measure=foundation.enum.MeasurementReference.difference
  Voltage Sensor : fl_lib/Electrical/Electrical Sensors/Voltage Sensor
  Voltage Sensor1 : fl_lib/Electrical/Electrical Sensors/Voltage Sensor
  gate_driver : Subsystem
  heatsink_C : fl_lib/Thermal/Thermal Elements/Thermal Mass  Commented=on  mass_type=foundation.enum.constant_variable.constant  mass=weigth/6 kg  sp_heat=cp_al J/(K*kg)  mass_min=1e-6 kg  num_ports=foundation.enum.numPorts2.one  m_specify=off  m_priority=High  m=1 kg  m_nominal_specify=off  m_nominal_value=1  m_nominal_unit=kg  T_specify=on  T_priority=High  T=DThs_init+Tambient degC  T_nominal_specify=off  T_nominal_value=1  T_nominal_unit=K  Q_specify=off  Q_priority=High  Q=0 W  Q_nominal_specify=off  Q_nominal_value=1  Q_nominal_unit=W
  heatsink_R : fl_lib/Thermal/Thermal Elements/Thermal Resistance  resistance=Rth_mosfet_HA K/W  T_specify=off  T_priority=High  T=0 deltadegC  T_nominal_specify=off  T_nominal_value=1  T_nominal_unit=K  Q_specify=off  Q_priority=None  Q=0 W  Q_nominal_specify=off  Q_nominal_value=1  Q_nominal_unit=W
  mosfet_sandwich : fl_lib/Thermal/Thermal Elements/Thermal Resistance  resistance=Rth_mosfet_JH K/W  T_specify=off  T_priority=High  T=0 degC  T_nominal_specify=off  T_nominal_value=1  T_nominal_unit=K  Q_specify=off  Q_priority=None  Q=0 W  Q_nominal_specify=off  Q_nominal_value=1  Q_nominal_unit=W
  power_losses_mosfet : Scope  Commented=on  NumInputPorts=2
      settings: SampleTime=tc  ActiveDisplayYMinimum=-6.15902  ActiveDisplayYMaximum=55.43118
  D : PMIOPort  Side=Left
  S : PMIOPort  Port=2  Side=Right
  tag scope: device_current_12=global, device_voltage_12=global, mosfet_12_power_losses=global, temperature_mosfet_12_HA=global, temperature_mosfet_12_JH=global, voltage_cm_device_12=global
  wires:
  PS-Simulink Converter/1 -> [mosfet_12_power_losses], power_losses_mosfet/1  "Power Losses"
  PS-Simulink Converter2/1 -> [temperature_mosfet_12_JH]  "mosfet_JH_temp"
  [temperature_mosfet_12_HA] -> Mux/2
  [temperature_mosfet_12_JH] -> Mux/1
  PS-Simulink Converter3/1 -> [temperature_mosfet_12_HA]  "mosfet_HA_temp"
  Mux/1 -> power_losses_mosfet/2
  PS-Simulink Converter1/1 -> [device_voltage_12]
  PS-Simulink Converter4/1 -> [device_current_12]
  PS-Simulink Converter5/1 -> [voltage_cm_device_12]
  G/1 -> gate_driver/1(cmd)
  connections:
  PS-Simulink Converter/LConn1 -- Heat Flow Rate Sensor/RConn1
  Voltage Sensor/RConn2 -- Voltage Sensor1/LConn1 -- Subsystem/RConn1 -- S/RConn1 -- gate_driver/RConn2
  Temperature Sensor/RConn2 -- PS-Simulink Converter2/LConn1
  Temperature Sensor1/RConn2 -- PS-Simulink Converter3/LConn1
  mosfet_sandwich/RConn1 -- heatsink_R/LConn1 -- heatsink_C/LConn1 -- Temperature Sensor/RConn1 -- Temperature Sensor1/LConn1
  Tambient/LConn1 -- heatsink_R/RConn1 -- Temperature Sensor1/RConn1
  Temperature Sensor/LConn1 -- mosfet_sandwich/LConn1 -- Heat Flow Rate Sensor/RConn2
  Voltage Sensor/RConn1 -- PS-Simulink Converter1/LConn1
  Current Sensor/LConn1 -- D/RConn1 -- Voltage Sensor/LConn1
  Lstray/LConn1 -- Current Sensor/RConn2
  Current Sensor/RConn1 -- PS-Simulink Converter4/LConn1
  PS-Simulink Converter5/LConn1 -- Voltage Sensor1/RConn1
  Voltage Sensor1/RConn2 -- Electrical Reference/LConn1
  Subsystem/LConn3 -- Lstray/RConn1
  Subsystem/LConn1 -- gate_driver/RConn1
  Heat Flow Rate Sensor/LConn1 -- Subsystem/LConn2

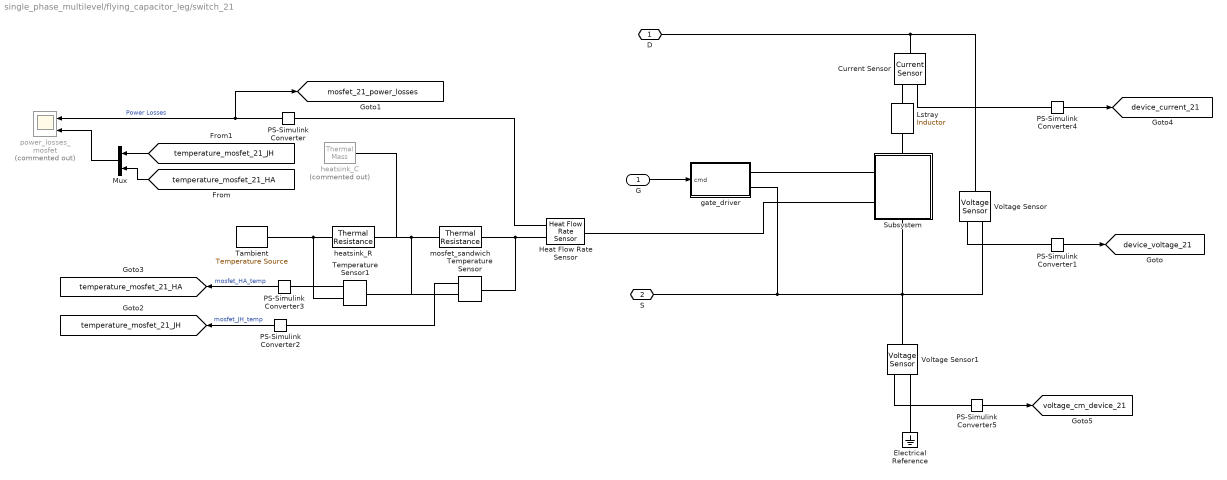
== system single_phase_multilevel/flying_capacitor_leg/switch_21 ==
  G : Inport
  Current Sensor : fl_lib/Electrical/Electrical Sensors/Current Sensor
  Electrical Reference : fl_lib/Electrical/Electrical Elements/Electrical Reference
  Heat Flow Rate Sensor : fl_lib/Thermal/Thermal Sensors/Heat Flow Rate Sensor
  Lstray : fl_lib/Electrical/Electrical Elements/Inductor  l=Lstray H  r=0 Ohm  g=1e-9 1/Ohm  i_specify=off  i_priority=None  i=0 A  i_nominal_specify=off  i_nominal_value=1  i_nominal_unit=A  v_specify=off  v_priority=None  v=0 V  v_nominal_specify=off  v_nominal_value=1  v_nominal_unit=V  i_L_specify=off  i_L_priority=High  i_L=0 A  i_L_nominal_specify=off  i_L_nominal_value=1  i_L_nominal_unit=A
  Mux : Mux  Inputs=2
  PS-Simulink Converter : nesl_utility/PS-Simulink Converter  PhysicalDomain=network_engine_domain  SubClassName=ps_output  LeftPortType=input  RightPortType=output  PseudoPeriodic=off  Frequencies=[]  VectorFormat=1-D array  Unit=W  AffineConversion=off
  PS-Simulink Converter1 : nesl_utility/PS-Simulink Converter  PhysicalDomain=network_engine_domain  SubClassName=ps_output  LeftPortType=input  RightPortType=output  PseudoPeriodic=off  Frequencies=[]  VectorFormat=1-D array  Unit=V  AffineConversion=off
  PS-Simulink Converter2 : nesl_utility/PS-Simulink Converter  PhysicalDomain=network_engine_domain  SubClassName=ps_output  LeftPortType=input  RightPortType=output  PseudoPeriodic=off  Frequencies=[]  VectorFormat=1-D array  Unit=degC  AffineConversion=off
  PS-Simulink Converter3 : nesl_utility/PS-Simulink Converter  PhysicalDomain=network_engine_domain  SubClassName=ps_output  LeftPortType=input  RightPortType=output  PseudoPeriodic=off  Frequencies=[]  VectorFormat=1-D array  Unit=degC  AffineConversion=off
  PS-Simulink Converter4 : nesl_utility/PS-Simulink Converter  PhysicalDomain=network_engine_domain  SubClassName=ps_output  LeftPortType=input  RightPortType=output  PseudoPeriodic=off  Frequencies=[]  VectorFormat=1-D array  Unit=A  AffineConversion=off
  PS-Simulink Converter5 : nesl_utility/PS-Simulink Converter  PhysicalDomain=network_engine_domain  SubClassName=ps_output  LeftPortType=input  RightPortType=output  PseudoPeriodic=off  Frequencies=[]  VectorFormat=1-D array  Unit=V  AffineConversion=off
  Subsystem : Subsystem
      settings: PortSchema="{\"entries\":[{\"content\":{\"sides\":[{\"content\":{\"connectorIds\":[\"LConn1\",\"LConn2\"]},\"type\":\"ConnectorPlacement.EquallySpacedRectSide\",\"uuid\":\"6f524266-aba9-462a-9d72-1145635a1e26\"},{\"content\":{\"side\":\"RIGHT\"},\"type\":\"ConnectorPlacement.EquallySpacedRectSide\",\"uuid\":\"542b2524-63ec-4375-9435-097c03e43763\"},{\"content\":{\"connectorIds\":[\"LConn3\"],\"side\":\"TOP\"},\"type\":\"ConnectorPlacement.EquallySpacedRectSide\",\"uuid\":\"19216a12-d28e-49a5-8583-2c9307a52e67\"},{\"content\":{\"connectorIds\":[\"RConn1\"],\"side\":\"BOTTOM\"},\"type\":\"ConnectorPlacement.EquallySpacedRectSide\",\"uuid\":\"0f3a6771-cb7b-4dcc-bba9-376db372f9ba\"}]},\"type\":\"ConnectorPlacement.EquallySpacedConnector\",\"uuid\":\"2de64d24-c5c0-4ec1-b56f-991356417e7b\"}],\"packageUris\":[\"http://schema.mathworks.com/mf0/Connector/R2020b\"],\"version\":\"1.0\"}"
  Tambient : fl_lib/Thermal/Thermal Sources/Temperature Source  temperature=Tambient degC
  Temperature Sensor : fl_lib/Thermal/Thermal Sensors/Temperature Sensor  temperature_measure=foundation.enum.MeasurementReference.difference
  Temperature Sensor1 : fl_lib/Thermal/Thermal Sensors/Temperature Sensor  temperature_measure=foundation.enum.MeasurementReference.difference
  Voltage Sensor : fl_lib/Electrical/Electrical Sensors/Voltage Sensor
  Voltage Sensor1 : fl_lib/Electrical/Electrical Sensors/Voltage Sensor
  gate_driver : Subsystem
  heatsink_C : fl_lib/Thermal/Thermal Elements/Thermal Mass  Commented=on  mass_type=foundation.enum.constant_variable.constant  mass=weigth/6 kg  sp_heat=cp_al J/(K*kg)  mass_min=1e-6 kg  num_ports=foundation.enum.numPorts2.one  m_specify=off  m_priority=High  m=1 kg  m_nominal_specify=off  m_nominal_value=1  m_nominal_unit=kg  T_specify=on  T_priority=High  T=DThs_init+Tambient degC  T_nominal_specify=off  T_nominal_value=1  T_nominal_unit=K  Q_specify=off  Q_priority=High  Q=0 W  Q_nominal_specify=off  Q_nominal_value=1  Q_nominal_unit=W
  heatsink_R : fl_lib/Thermal/Thermal Elements/Thermal Resistance  resistance=Rth_mosfet_HA K/W  T_specify=off  T_priority=High  T=0 deltadegC  T_nominal_specify=off  T_nominal_value=1  T_nominal_unit=K  Q_specify=off  Q_priority=None  Q=0 W  Q_nominal_specify=off  Q_nominal_value=1  Q_nominal_unit=W
  mosfet_sandwich : fl_lib/Thermal/Thermal Elements/Thermal Resistance  resistance=Rth_mosfet_JH K/W  T_specify=off  T_priority=High  T=0 degC  T_nominal_specify=off  T_nominal_value=1  T_nominal_unit=K  Q_specify=off  Q_priority=None  Q=0 W  Q_nominal_specify=off  Q_nominal_value=1  Q_nominal_unit=W
  power_losses_mosfet : Scope  Commented=on  NumInputPorts=2
      settings: SampleTime=tc  ActiveDisplayYMinimum=-6.15902  ActiveDisplayYMaximum=55.43118
  D : PMIOPort  Side=Left
  S : PMIOPort  Port=2  Side=Right
  tag scope: device_current_21=global, device_voltage_21=global, mosfet_21_power_losses=global, temperature_mosfet_21_HA=global, temperature_mosfet_21_JH=global, voltage_cm_device_21=global
  wires:
  PS-Simulink Converter/1 -> [mosfet_21_power_losses], power_losses_mosfet/1  "Power Losses"
  PS-Simulink Converter2/1 -> [temperature_mosfet_21_JH]  "mosfet_JH_temp"
  [temperature_mosfet_21_HA] -> Mux/2
  [temperature_mosfet_21_JH] -> Mux/1
  PS-Simulink Converter3/1 -> [temperature_mosfet_21_HA]  "mosfet_HA_temp"
  Mux/1 -> power_losses_mosfet/2
  PS-Simulink Converter1/1 -> [device_voltage_21]
  PS-Simulink Converter4/1 -> [device_current_21]
  PS-Simulink Converter5/1 -> [voltage_cm_device_21]
  G/1 -> gate_driver/1(cmd)
  connections:
  PS-Simulink Converter/LConn1 -- Heat Flow Rate Sensor/RConn1
  Voltage Sensor/RConn2 -- Subsystem/RConn1 -- gate_driver/RConn2 -- S/RConn1 -- Voltage Sensor1/LConn1
  Temperature Sensor/RConn2 -- PS-Simulink Converter2/LConn1
  Temperature Sensor1/RConn2 -- PS-Simulink Converter3/LConn1
  mosfet_sandwich/RConn1 -- heatsink_C/LConn1 -- heatsink_R/LConn1 -- Temperature Sensor/RConn1 -- Temperature Sensor1/LConn1
  Tambient/LConn1 -- heatsink_R/RConn1 -- Temperature Sensor1/RConn1
  Temperature Sensor/LConn1 -- mosfet_sandwich/LConn1 -- Heat Flow Rate Sensor/RConn2
  Voltage Sensor/RConn1 -- PS-Simulink Converter1/LConn1
  Current Sensor/LConn1 -- D/RConn1 -- Voltage Sensor/LConn1
  Lstray/LConn1 -- Current Sensor/RConn2
  Current Sensor/RConn1 -- PS-Simulink Converter4/LConn1
  PS-Simulink Converter5/LConn1 -- Voltage Sensor1/RConn1
  Voltage Sensor1/RConn2 -- Electrical Reference/LConn1
  Subsystem/LConn3 -- Lstray/RConn1
  Heat Flow Rate Sensor/LConn1 -- Subsystem/LConn2
  gate_driver/RConn1 -- Subsystem/LConn1

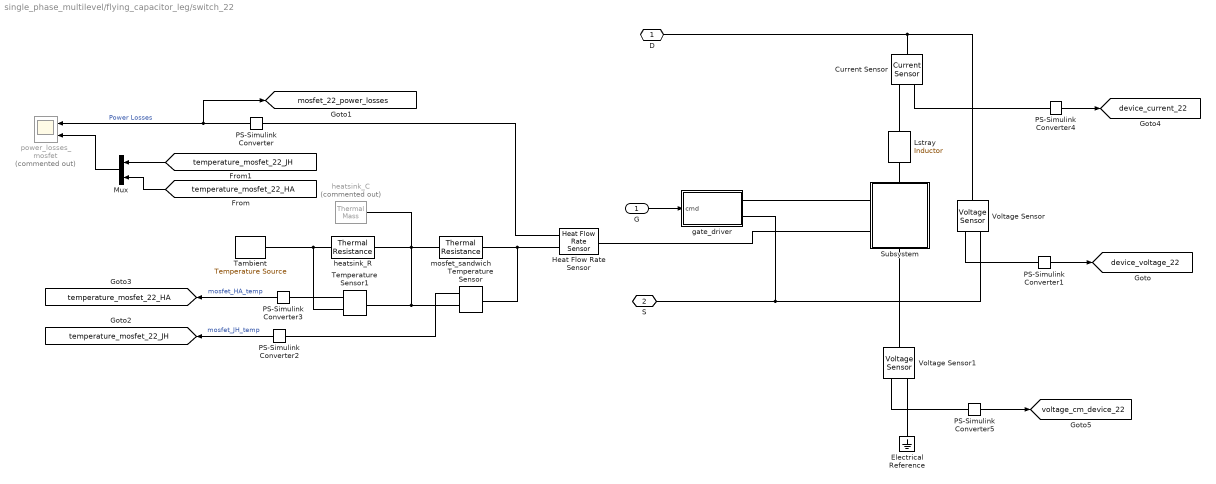
== system single_phase_multilevel/flying_capacitor_leg/switch_22 ==
  G : Inport
  Current Sensor : fl_lib/Electrical/Electrical Sensors/Current Sensor
  Electrical Reference : fl_lib/Electrical/Electrical Elements/Electrical Reference
  Heat Flow Rate Sensor : fl_lib/Thermal/Thermal Sensors/Heat Flow Rate Sensor
  Lstray : fl_lib/Electrical/Electrical Elements/Inductor  l=Lstray H  r=0 Ohm  g=1e-9 1/Ohm  i_specify=off  i_priority=None  i=0 A  i_nominal_specify=off  i_nominal_value=1  i_nominal_unit=A  v_specify=off  v_priority=None  v=0 V  v_nominal_specify=off  v_nominal_value=1  v_nominal_unit=V  i_L_specify=off  i_L_priority=High  i_L=0 A  i_L_nominal_specify=off  i_L_nominal_value=1  i_L_nominal_unit=A
  Mux : Mux  Inputs=2
  PS-Simulink Converter : nesl_utility/PS-Simulink Converter  PhysicalDomain=network_engine_domain  SubClassName=ps_output  LeftPortType=input  RightPortType=output  PseudoPeriodic=off  Frequencies=[]  VectorFormat=1-D array  Unit=W  AffineConversion=off
  PS-Simulink Converter1 : nesl_utility/PS-Simulink Converter  PhysicalDomain=network_engine_domain  SubClassName=ps_output  LeftPortType=input  RightPortType=output  PseudoPeriodic=off  Frequencies=[]  VectorFormat=1-D array  Unit=V  AffineConversion=off
  PS-Simulink Converter2 : nesl_utility/PS-Simulink Converter  PhysicalDomain=network_engine_domain  SubClassName=ps_output  LeftPortType=input  RightPortType=output  PseudoPeriodic=off  Frequencies=[]  VectorFormat=1-D array  Unit=degC  AffineConversion=off
  PS-Simulink Converter3 : nesl_utility/PS-Simulink Converter  PhysicalDomain=network_engine_domain  SubClassName=ps_output  LeftPortType=input  RightPortType=output  PseudoPeriodic=off  Frequencies=[]  VectorFormat=1-D array  Unit=degC  AffineConversion=off
  PS-Simulink Converter4 : nesl_utility/PS-Simulink Converter  PhysicalDomain=network_engine_domain  SubClassName=ps_output  LeftPortType=input  RightPortType=output  PseudoPeriodic=off  Frequencies=[]  VectorFormat=1-D array  Unit=A  AffineConversion=off
  PS-Simulink Converter5 : nesl_utility/PS-Simulink Converter  PhysicalDomain=network_engine_domain  SubClassName=ps_output  LeftPortType=input  RightPortType=output  PseudoPeriodic=off  Frequencies=[]  VectorFormat=1-D array  Unit=V  AffineConversion=off
  Subsystem : Subsystem
      settings: PortSchema="{\"entries\":[{\"content\":{\"sides\":[{\"content\":{\"connectorIds\":[\"LConn1\",\"LConn2\"]},\"type\":\"ConnectorPlacement.EquallySpacedRectSide\",\"uuid\":\"6f524266-aba9-462a-9d72-1145635a1e26\"},{\"content\":{\"side\":\"RIGHT\"},\"type\":\"ConnectorPlacement.EquallySpacedRectSide\",\"uuid\":\"542b2524-63ec-4375-9435-097c03e43763\"},{\"content\":{\"connectorIds\":[\"LConn3\"],\"side\":\"TOP\"},\"type\":\"ConnectorPlacement.EquallySpacedRectSide\",\"uuid\":\"19216a12-d28e-49a5-8583-2c9307a52e67\"},{\"content\":{\"connectorIds\":[\"RConn1\"],\"side\":\"BOTTOM\"},\"type\":\"ConnectorPlacement.EquallySpacedRectSide\",\"uuid\":\"0f3a6771-cb7b-4dcc-bba9-376db372f9ba\"}]},\"type\":\"ConnectorPlacement.EquallySpacedConnector\",\"uuid\":\"2de64d24-c5c0-4ec1-b56f-991356417e7b\"}],\"packageUris\":[\"http://schema.mathworks.com/mf0/Connector/R2020b\"],\"version\":\"1.0\"}"
  Tambient : fl_lib/Thermal/Thermal Sources/Temperature Source  temperature=Tambient degC
  Temperature Sensor : fl_lib/Thermal/Thermal Sensors/Temperature Sensor  temperature_measure=foundation.enum.MeasurementReference.difference
  Temperature Sensor1 : fl_lib/Thermal/Thermal Sensors/Temperature Sensor  temperature_measure=foundation.enum.MeasurementReference.difference
  Voltage Sensor : fl_lib/Electrical/Electrical Sensors/Voltage Sensor
  Voltage Sensor1 : fl_lib/Electrical/Electrical Sensors/Voltage Sensor
  gate_driver : Subsystem
  heatsink_C : fl_lib/Thermal/Thermal Elements/Thermal Mass  Commented=on  mass_type=foundation.enum.constant_variable.constant  mass=weigth/6 kg  sp_heat=cp_al J/(K*kg)  mass_min=1e-6 kg  num_ports=foundation.enum.numPorts2.one  m_specify=off  m_priority=High  m=1 kg  m_nominal_specify=off  m_nominal_value=1  m_nominal_unit=kg  T_specify=on  T_priority=High  T=DThs_init+Tambient degC  T_nominal_specify=off  T_nominal_value=1  T_nominal_unit=K  Q_specify=off  Q_priority=High  Q=0 W  Q_nominal_specify=off  Q_nominal_value=1  Q_nominal_unit=W
  heatsink_R : fl_lib/Thermal/Thermal Elements/Thermal Resistance  resistance=Rth_mosfet_HA K/W  T_specify=off  T_priority=High  T=0 deltadegC  T_nominal_specify=off  T_nominal_value=1  T_nominal_unit=K  Q_specify=off  Q_priority=None  Q=0 W  Q_nominal_specify=off  Q_nominal_value=1  Q_nominal_unit=W
  mosfet_sandwich : fl_lib/Thermal/Thermal Elements/Thermal Resistance  resistance=Rth_mosfet_JH K/W  T_specify=off  T_priority=High  T=0 degC  T_nominal_specify=off  T_nominal_value=1  T_nominal_unit=K  Q_specify=off  Q_priority=None  Q=0 W  Q_nominal_specify=off  Q_nominal_value=1  Q_nominal_unit=W
  power_losses_mosfet : Scope  Commented=on  NumInputPorts=2
      settings: SampleTime=tc  ActiveDisplayYMinimum=-6.15902  ActiveDisplayYMaximum=55.43118
  D : PMIOPort  Side=Left
  S : PMIOPort  Port=2  Side=Right
  tag scope: device_current_22=global, device_voltage_22=global, mosfet_22_power_losses=global, temperature_mosfet_22_HA=global, temperature_mosfet_22_JH=global, voltage_cm_device_22=global
  wires:
  PS-Simulink Converter1/1 -> [device_voltage_22]
  Mux/1 -> power_losses_mosfet/2
  PS-Simulink Converter3/1 -> [temperature_mosfet_22_HA]  "mosfet_HA_temp"
  [temperature_mosfet_22_JH] -> Mux/1
  [temperature_mosfet_22_HA] -> Mux/2
  PS-Simulink Converter2/1 -> [temperature_mosfet_22_JH]  "mosfet_JH_temp"
  PS-Simulink Converter/1 -> power_losses_mosfet/1, [mosfet_22_power_losses]  "Power Losses"
  PS-Simulink Converter4/1 -> [device_current_22]
  PS-Simulink Converter5/1 -> [voltage_cm_device_22]
  G/1 -> gate_driver/1(cmd)
  connections:
  Voltage Sensor/RConn1 -- PS-Simulink Converter1/LConn1
  Heat Flow Rate Sensor/RConn2 -- mosfet_sandwich/LConn1 -- Temperature Sensor/LConn1
  Temperature Sensor1/RConn1 -- heatsink_R/RConn1 -- Tambient/LConn1
  Temperature Sensor1/LConn1 -- Temperature Sensor/RConn1 -- heatsink_R/LConn1 -- heatsink_C/LConn1 -- mosfet_sandwich/RConn1
  Temperature Sensor1/RConn2 -- PS-Simulink Converter3/LConn1
  Temperature Sensor/RConn2 -- PS-Simulink Converter2/LConn1
  Subsystem/RConn1 -- Voltage Sensor/RConn2 -- Voltage Sensor1/LConn1 -- gate_driver/RConn2 -- S/RConn1
  PS-Simulink Converter/LConn1 -- Heat Flow Rate Sensor/RConn1
  Current Sensor/LConn1 -- D/RConn1 -- Voltage Sensor/LConn1
  Lstray/LConn1 -- Current Sensor/RConn2
  Current Sensor/RConn1 -- PS-Simulink Converter4/LConn1
  PS-Simulink Converter5/LConn1 -- Voltage Sensor1/RConn1
  Voltage Sensor1/RConn2 -- Electrical Reference/LConn1
  Subsystem/LConn3 -- Lstray/RConn1
  Subsystem/LConn1 -- gate_driver/RConn1
  Heat Flow Rate Sensor/LConn1 -- Subsystem/LConn2
